simulink model "MPC_Prototyping_Ship_Control"  (R2024a)
settings: Solver=VariableStepAuto  StartTime=0.0  StopTime=8  RelTol=1e-3
values from neighbouring files (symbols this model uses):
  Input_Matrix_Ship_Nominal = [0;Time_Sampling*(Static_Gain_Ship_Nominal/Time_Constant_Ship_Nominal)]    [Model_Predictive_Control_Prototyping.m]
  Input_Measurement_Matrix_Ship_Nominal = [0;0]    [Model_Predictive_Control_Prototyping.m]
  Measurement_Matrix_Ship_Nominal = [1 0;0 1]    [Model_Predictive_Control_Prototyping.m]
  State_Matrix_Ship_Nominal = [1 Time_Sampling ... (first row only)    [Model_Predictive_Control_Prototyping.m]
settings Model: Creator=gerar  LastModifiedBy=gerar

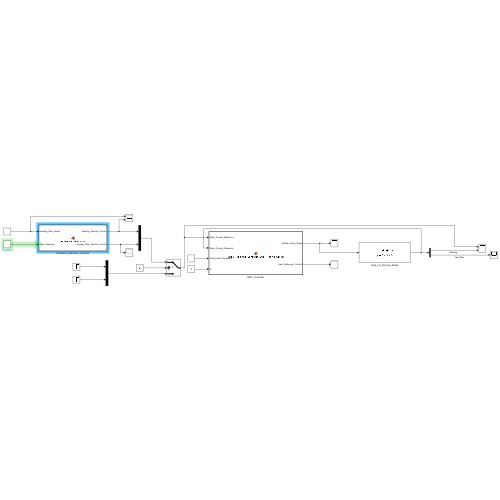
[thumbnail: Simulink's stored preview of the top-level diagram]
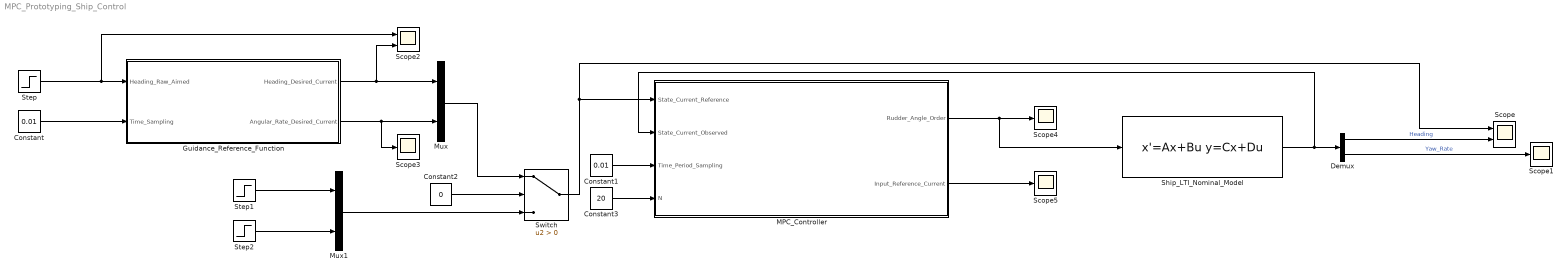
== system MPC_Prototyping_Ship_Control ==
  Constant : Constant  Value=0.01
  Constant1 : Constant  Value=0.01
  Constant2 : Constant  Value=0
  Constant3 : Constant  Value=20
  Demux : Demux  Outputs=2
  Guidance_Reference_Function : MATLAB Function  TreatAsAtomicUnit=on  SystemSampleTime=0.01
  MPC_Controller : MATLAB Function  TreatAsAtomicUnit=on  SystemSampleTime=0.01
  Mux : Mux  Inputs=2
  Mux1 : Mux  Inputs=2
  Scope : Scope  NumInputPorts=2
  Scope{1,3..5} (4 alike) : Scope
  Scope2 : Scope  NumInputPorts=2
  Ship_LTI_Nominal_Model : StateSpace  A=State_Matrix_Ship_Nominal  B=Input_Matrix_Ship_Nominal  C=Measurement_Matrix_Ship_Nominal  D=Input_Measurement_Matrix_Ship_Nominal  InitialCondition=0
  Step : Step  After=30*(pi/180)  SampleTime=0
  Step1 : Step  Time=0  After=30*(pi/180)  SampleTime=0
  Step2 : Step  Time=0  After=15*(pi/180)  SampleTime=0
  Switch : Switch  Criteria=u2 > Threshold  SaturateOnIntegerOverflow=off  InputSameDT=off
  wires:
  Ship_LTI_Nominal_Model/1 -> MPC_Controller/2(State_Current_Observed), Demux/1
  Demux/1 -> Scope/2  "Heading"
  Demux/2 -> Scope1/1  "Yaw_Rate"
  Step/1 -> Scope2/1, Guidance_Reference_Function/1(Heading_Raw_Aimed)
  Constant/1 -> Guidance_Reference_Function/2(Time_Sampling)
  Guidance_Reference_Function/1(Heading_Desired_Current) -> Scope2/2, Mux/1
  Guidance_Reference_Function/2(Angular_Rate_Desired_Current) -> Scope3/1, Mux/2
  Mux/1 -> Switch/1
  Constant1/1 -> MPC_Controller/3(Time_Period_Sampling)
  MPC_Controller/2(Input_Reference_Current) -> Scope5/1
  MPC_Controller/1(Rudder_Angle_Order) -> Scope4/1, Ship_LTI_Nominal_Model/1
  Step1/1 -> Mux1/1
  Step2/1 -> Mux1/2
  Mux1/1 -> Switch/3
  Constant2/1 -> Switch/2
  Switch/1 -> MPC_Controller/1(State_Current_Reference), Scope/1
  Constant3/1 -> MPC_Controller/4(N)

== matlab function MPC_Prototyping_Ship_Control/MPC_Controller ==
  data: State_Current_Reference input; State_Current_Observed input; Rudder_Angle_Order output; Time_Period_Sampling input; Input_Reference_Current output; N input
function [Rudder_Angle_Order,Input_Reference_Current] = Model_Predictive_Controller_Ship_Heading_Control(State_Current_Reference,...
                                                                                                         State_Current_Observed,...
                                                                                                         Time_Period_Sampling,...
                                                                                                         N)

% % Initialization parameters for the embedded ship model:
% Static_Gain_Ship_Nominal = 0.6043;
% Time_Constant_Ship_Nominal = -5.2097;
% Time_Sampling = Time_Period_Sampling;
% State_Matrix_Ship_Nominal = [1 Time_Sampling;
%                              0 1-(Time_Sampling/Time_Constant_Ship_Nominal)];
% Input_Matrix_Ship_Nominal = [0;Time_Sampling*(Static_Gain_Ship_Nominal/Time_Constant_Ship_Nominal)];
% Measurement_Matrix_Ship_Nominal = [1 0;0 1];
% Input_Measurement_Matrix_Ship_Nominal = [0;0];
% 
% % Reference input:
% % Input_Reference_Current = (Input_Matrix_Ship_Nominal\(eye(2) - State_Matrix_Ship_Nominal))*State_Current_Reference;
% Input_Reference_Current = pinv(Input_Matrix_Ship_Nominal)*(eye(2) - State_Matrix_Ship_Nominal)*State_Current_Reference;
% 
% % Parametrization of the embedded model:
% % Note that the following augmented model is based on the fact that the
% % choice has been made to take a prediction horizon of 3. Hence the shape
% % of the augmented matrices of the system.
% Weight_State_1_Heading = 0.1;
% Weight_State_2_Yaw_Rate = 10;
% Weight_Input_Rudder_Angle = 100;
% State_Matrix_Weight_Penalization = [Weight_State_1_Heading 0;
%                                     0 Weight_State_2_Yaw_Rate];
% % Final state penalization:
% Weight_State_1_Final_Heading = 0.1;
% Weight_State_2_Final_Yaw_Rate = 10;
% State_Matrix_Weight_Penalization_Final = [Weight_State_1_Final_Heading 0;
%                                           0 Weight_State_2_Final_Yaw_Rate];
% % Input state penalization:
% Input_Matrix_Weight_Penalization = Weight_Input_Rudder_Angle;
% % Augmented weight matrices:
% State_Matrix_Weight_Penalization_Augmented = [State_Matrix_Weight_Penalization zeros(2,2) zeros(2,2) zeros(2,2);
%                                               zeros(2,2) State_Matrix_Weight_Penalization zeros(2,2) zeros(2,2);
%                                               zeros(2,2) zeros(2,2) State_Matrix_Weight_Penalization zeros(2,2);
%                                               zeros(2,2) zeros(2,2) zeros(2,2) State_Matrix_Weight_Penalization_Final];
% Input_Matrix_Weight_Penalization_Augmented = [Input_Matrix_Weight_Penalization 0 0;
%                                               0 Input_Matrix_Weight_Penalization 0;
%                                               0 0 Input_Matrix_Weight_Penalization];
% Input_Matrix_Augmented_System = [zeros(2,1) zeros(2,1) zeros(2,1);
%                                  Input_Matrix_Ship_Nominal zeros(2,1) zeros(2,1);
%                                  State_Matrix_Ship_Nominal*Input_Matrix_Ship_Nominal Input_Matrix_Ship_Nominal zeros(2,1);
%                                  State_Matrix_Ship_Nominal^2*Input_Matrix_Ship_Nominal State_Matrix_Ship_Nominal*Input_Matrix_Ship_Nominal Input_Matrix_Ship_Nominal];
% State_Matrix_Augmented_System = [eye(2);
%                                  State_Matrix_Ship_Nominal;
%                                  State_Matrix_Ship_Nominal^2;
%                                  State_Matrix_Ship_Nominal^3];
% Matrix_Cost_Function_Optimizator = [State_Matrix_Weight_Penalization_Augmented zeros(8,3);
%                                     zeros(3,8) Input_Matrix_Weight_Penalization_Augmented];
% % Equality constraint functions for the optimization:
% Function_Equality_Constraint = [eye(8) -Input_Matrix_Augmented_System];
% State_Vector_Error_Current = State_Current_Observed - State_Current_Reference;
% Equality_Contraint = State_Matrix_Augmented_System*State_Vector_Error_Current;
% % Inequality contraint functions definition:
% Rudder_Rate_Maximal = 10*(pi/180);
% Rudder_Rate_Minimal = -10*(pi/180);
% Heading_Maximal = pi;
% Heading_Minimal = -pi;
% Function_Inequality_Constraint_State_Classical = [1 0;
%                                                   -1 0;
%                                                   0 1;
%                                                   0 -1];
% Inequality_Constraint_State_Classical = [Heading_Maximal;-Heading_Minimal;Rudder_Rate_Maximal;-Rudder_Rate_Minimal];
% Function_Inequality_Constraint_State_Augmented = [Function_Inequality_Constraint_State_Classical zeros(4,2) zeros(4,2) zeros(4,2);
%                                                   zeros(4,2) Function_Inequality_Constraint_State_Classical zeros(4,2) zeros(4,2);
%                                                   zeros(4,2) zeros(4,2) Function_Inequality_Constraint_State_Classical zeros(4,2);
%                                                   zeros(4,2) zeros(4,2) zeros(4,2) Function_Inequality_Constraint_State_Classical];
% Inequality_Constraint_State_Augmented = [Inequality_Constraint_State_Classical;Inequality_Constraint_State_Classical;Inequality_Constraint_State_Classical;Inequality_Constraint_State_Classical];
% Inequality_Constraint_State_Augmented_Reference = [Inequality_Constraint_State_Classical - Function_Inequality_Constraint_State_Classical*State_Current_Reference;
%                                                    Inequality_Constraint_State_Classical - Function_Inequality_Constraint_State_Classical*State_Current_Reference;
%                                                    Inequality_Constraint_State_Classical - Function_Inequality_Constraint_State_Classical*State_Current_Reference;
%                                                    Inequality_Constraint_State_Classical - Function_Inequality_Constraint_State_Classical*State_Current_Reference;];
% Rudder_Angle_Maximal = 35*(pi/180);
% Rudder_Angle_Minimal = -35*(pi/180);
% Function_Inequality_Constraint_Input_Classical = [1;-1];
% Inequality_Constraint_Input_Classical = [Rudder_Angle_Maximal;-Rudder_Angle_Minimal];
% Function_Inequality_Constraint_Input_Augmented = [Function_Inequality_Constraint_Input_Classical zeros(2,1) zeros(2,1);
%                                                   zeros(2,1) Function_Inequality_Constraint_Input_Classical zeros(2,1);
%                                                   zeros(2,1) zeros(2,1) Function_Inequality_Constraint_Input_Classical];
% Inequality_Constraint_Input_Augmented = [Inequality_Constraint_Input_Classical;Inequality_Constraint_Input_Classical;Inequality_Constraint_Input_Classical];
% Inequality_Constraint_Input_Augmented_Reference = [Inequality_Constraint_Input_Classical - Function_Inequality_Constraint_Input_Classical*Input_Reference_Current;
%                                                    Inequality_Constraint_Input_Classical - Function_Inequality_Constraint_Input_Classical*Input_Reference_Current;
%                                                    Inequality_Constraint_Input_Classical - Function_Inequality_Constraint_Input_Classical*Input_Reference_Current];
% % State and input augmented inequality constraint functions:
% Function_Inequality_Constraint_State_Input = [Function_Inequality_Constraint_State_Augmented zeros(16,3);
%                                               zeros(6,8) Function_Inequality_Constraint_Input_Augmented];
% Inequality_Consrtaint_State_Input = [Inequality_Constraint_State_Augmented_Reference;
%                                      Inequality_Constraint_Input_Augmented_Reference];
% 
% % Optimization problem solving:
% State_Vector_Initial = [35*(pi/180);0];
% Input_Vector_Initial = 0;
% State_Input_Vector_Error_Initial = [State_Vector_Initial - State_Current_Reference;
%                                     State_Vector_Initial - State_Current_Reference;
%                                     State_Vector_Initial - State_Current_Reference;
%                                     State_Vector_Initial - State_Current_Reference;
%                                     Input_Vector_Initial - Input_Reference_Current;
%                                     Input_Vector_Initial - Input_Reference_Current;
%                                     Input_Vector_Initial - Input_Reference_Current];
% Optimization_Options = optimoptions("quadprog","Algorithm","active-set","Display","none");
% Cost_Function_Second = zeros(1,11);
% Normalized_Matrix_Cost_Function = (Matrix_Cost_Function_Optimizator + Matrix_Cost_Function_Optimizator')/2;
% Normalized_Matrix_Cost_Function = Normalized_Matrix_Cost_Function + 1e-6 * eye(size(Normalized_Matrix_Cost_Function));
% [Vector_Optimization,~,Exit_Flag] = quadprog(Normalized_Matrix_Cost_Function,...
%                                              Cost_Function_Second,...
%                                              Function_Inequality_Constraint_State_Input,...
%                                              Inequality_Consrtaint_State_Input,...
%                                              Function_Equality_Constraint,...
%                                              Equality_Contraint,...
%                                              [],...
%                                              [],...
%                                              State_Input_Vector_Error_Initial,...
%                                              Optimization_Options);
% 
% % Use of another optimizer:
% Optimal_Rudder_Angle_Vector = Vector_Optimization(9:end);
% Optimal_Rudder_First_Action = Optimal_Rudder_Angle_Vector(1);
% Rudder_Angle_Order = Optimal_Rudder_First_Action + Input_Reference_Current;
%% --- Model Parameters ---
K_ship = 0.6043;
T_ship = -5.2097;   % stays negative (as per your identified model)
Ts = Time_Period_Sampling;

A = [1, Ts;
     0, 1 - Ts/T_ship];
B = [0; Ts*(K_ship/T_ship)];

%% --- Reference Input ---
Input_Reference_Current = pinv(B)*(eye(2) - A)*State_Current_Reference;

%% --- Weight Matrices ---
Q = diag([0.1, 10]);
Qf = diag([0.1, 10]);
R = 100;

%% --- Build Augmented Matrices for Horizon N ---
n = size(A,1);
m = size(B,2);

Phi = zeros(N*n, n);
Gamma = zeros(N*n, N*m);

for i = 1:N
    Phi((i-1)*n+1:i*n, :) = A^i;
    for j = 1:i
        Gamma((i-1)*n+1:i*n, (j-1)*m+1:j*m) = A^(i-j)*B;
    end
end

%% --- Cost Matrices (Quadratic form) ---
Qbar = kron(eye(N), Q);
Qbar(end-n+1:end, end-n+1:end) = Qf; % final weight
Rbar = kron(eye(N), R);
H = blkdiag(Qbar, Rbar);
% H = (H + H')/2 + 1e-8*eye(size(H)); % regularization
H = 2*H;

%% --- Equality Constraints (dynamics) ---
Feq = [eye(N*n), -Gamma];
beq = Phi * (State_Current_Observed - State_Current_Reference);

%% --- Inequality Constraints ---
Heading_Max = pi;
Heading_Min = -pi;
YawRate_Max = 10*pi/180;
YawRate_Min = -10*pi/180;

Fx_block = [1 0; -1 0; 0 1; 0 -1];
gx_block = [Heading_Max; -Heading_Min; YawRate_Max; -YawRate_Min];

Fx = kron(eye(N), Fx_block);
gx = repmat(gx_block, N, 1);

Rudder_Max = 35*pi/180;
Rudder_Min = -35*pi/180;
Fu_block = [1; -1];
gu_block = [Rudder_Max; -Rudder_Min];

Fu = kron(eye(N), Fu_block);
gu = repmat(gu_block, N, 1);

% Combine constraints
Fineq = blkdiag(Fx, Fu);
gineq = [gx; gu];

%% --- Solve QP ---
f = zeros(size(H,1),1);
x0 = zeros(size(H,1),1);

opts = optimoptions('quadprog','Algorithm','active-set','Display','off');
[z_opt, ~, exitflag] = quadprog(H, f, Fineq, gineq, Feq, beq, [], [], x0, opts);

if exitflag ~= 1
    warning('quadprog did not converge. Exitflag=%d', exitflag);
end

%% --- Extract Control Command ---
U_opt = z_opt(N*n+1:end);
u_e_k = U_opt(1);
Rudder_Angle_Order = u_e_k + Input_Reference_Current;

end

== matlab function MPC_Prototyping_Ship_Control/Guidance_Reference_Function ==
  data: Heading_Raw_Aimed input; Heading_Desired_Current output; Time_Sampling input; Angular_Rate_Desired_Current output
function [Heading_Desired_Current,Angular_Rate_Desired_Current] = Reference_To_Desired(Heading_Raw_Aimed,Time_Sampling)

% Initialization:
% Persistents for reference model used:
persistent Angular_Acceleration_Desired_Previous;
persistent Rudder_Rate_Desired_Previous;
persistent Heading_Desired_Previous;
persistent Heading_Aimed_Previous_Raw;
if isempty(Heading_Desired_Previous)
    Heading_Desired_Previous = 0;
    Rudder_Rate_Desired_Previous = 0;
    Angular_Acceleration_Desired_Previous = 0;
    Heading_Aimed_Previous_Raw = 0;
end
Rudder_Rate_Saturation = 10*(pi/180);
Rudder_Acceleration_Saturation = 10*(pi/180);
Damping_Reference_Model = 1; % Smooth.
Pulsation_Reference_Model = 0.5; % Smaller thant the one of the closed-loop bandwidth.

Jerk_Desired_Current = -(2*Damping_Reference_Model + 1)*Pulsation_Reference_Model*Angular_Acceleration_Desired_Previous - (2*Damping_Reference_Model + 1)*Pulsation_Reference_Model^2*...
                       Rudder_Rate_Desired_Previous + Pulsation_Reference_Model^3*(Heading_Aimed_Previous_Raw - Heading_Desired_Previous);
Angular_Acceleration_Desired_Current = Angular_Acceleration_Desired_Previous + Time_Sampling*Jerk_Desired_Current;
% Saturation:
Angular_Acceleration_Desired_Current = max(min(Angular_Acceleration_Desired_Current, Rudder_Acceleration_Saturation), -Rudder_Acceleration_Saturation);

% Angular rate iteration:
% Angular_Rate_Desired_Current = Rudder_Rate_Desired_Previous + Time_Sampling*Acceleration_Desired_Previous;
Angular_Rate_Desired_Current = Rudder_Rate_Desired_Previous + Time_Sampling*Angular_Acceleration_Desired_Current;
% Saturation:
Angular_Rate_Desired_Current = max(min(Angular_Rate_Desired_Current, Rudder_Rate_Saturation), -Rudder_Rate_Saturation);

% Heading desired:
% Heading_Desired_Current = Heading_Desired_Previous + Time_Sampling*Rate_Desired_Previous;
Heading_Desired_Current = Heading_Desired_Previous + Time_Sampling*Angular_Rate_Desired_Current;

% Persistent update:
Heading_Aimed_Previous_Raw = Heading_Raw_Aimed;
Rudder_Rate_Desired_Previous = Angular_Rate_Desired_Current;
Angular_Acceleration_Desired_Previous = Angular_Acceleration_Desired_Current;
Heading_Desired_Previous = Heading_Desired_Current;


end
